simulink model "SISO_Sim_a"  (R2015b)
settings: Solver=VariableStepAuto  StartTime=0.0  StopTime=15  RelTol=1e-3
libraries: simulink_extras x2, simulink x1
settings Model: Creator=dmartin_a  LastModifiedBy=dmartin_a

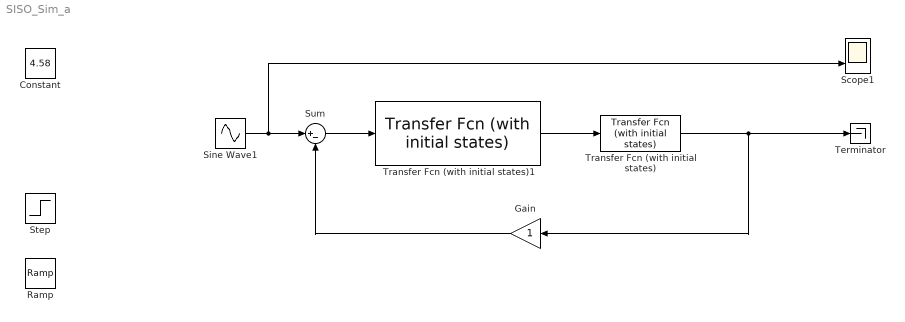
== system SISO_Sim_a ==
  Constant : Constant  Value=4.58
  Gain : Gain
  Ramp : simulink/Sources/Ramp  slope=2  start=5  X0=0
  Scope1 : Scope  NumInputPorts=2
  Sine Wave1 : Sin  SampleTime=0
  Step : Step  SampleTime=0
  Sum : Sum  Inputs=|+-
  Terminator : Terminator
  Transfer Fcn (with initial states) : simulink_extras/Additional Linear/Transfer Fcn (with initial states)  N=[31.62 -0.1]  D="[1  -24.4 0 0]"  X0=2
  Transfer Fcn (with initial states)1 : simulink_extras/Additional Linear/Transfer Fcn (with initial states)  N=[3.248e4 -3.1625e4 -1e4]  D=[1 524.3984 -1.02e4]  X0=1
  wires:
  Transfer Fcn (with initial states)1/1 -> Transfer Fcn (with initial states)/1
  Sum/1 -> Transfer Fcn (with initial states)1/1
  Transfer Fcn (with initial states)/1 -> Terminator/1, Gain/1
  Gain/1 -> Sum/2
  Sine Wave1/1 -> Scope1/2, Sum/1
